simulink model "atti"  (R2022b)
settings: Solver=VariableStepAuto  StartTime=0.0  StopTime=10.0  RelTol=1e-3
values from neighbouring files (symbols this model uses):
  dt = 0.01    [attitude_main.m]
  dtheta = [x;y;z]'    [attitude_main.m]
  J = diag([0.082,0.0845,0.1377])    [attitude_main.m]
  K = lqr(sys,Q,R)    [attitude_main.m]
undefined symbols (not defined in the file or in its folder): ad, Rd, wd
libraries: shared6dof x1, aerolibutil x1
settings Model: Creator=zzy  LastModifiedBy=zzy
settings DataIOCC: ReturnWorkspaceOutputs=off

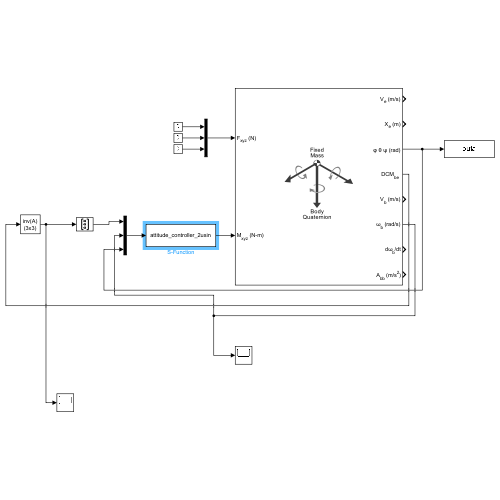
[thumbnail: Simulink's stored preview of the top-level diagram]
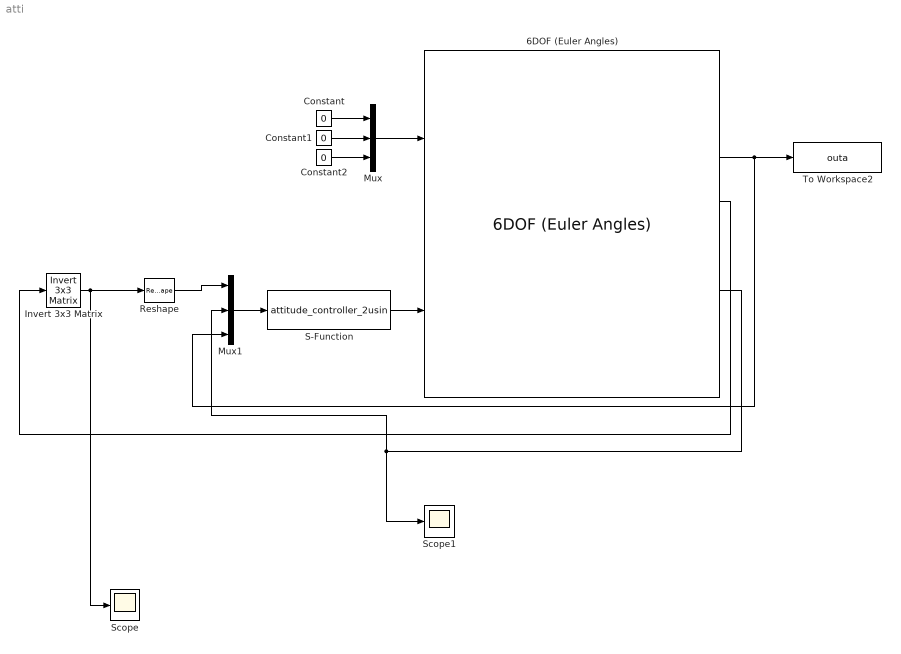
== system atti ==
  6DOF (Euler Angles) : shared6dof/6DOF (Euler Angles)  units=Metric (MKS)  mtype=Fixed  rep=Quaternion  xme_0=[0 0 0]  Vm_0=[0 0 0]  eul_0=[0 0 0]  pm_0=[0 0 0]  mass_0=1  mass_e=0.5  mass_f=2.0  inertia=J  inertia_e=eye(3)  inertia_f=2*eye(3)  k_quat=1.0  vre_flag=on  abi_flag=off  aMode=0  xme_statename=''  Vm_statename=''  eul_statename=''  quat_statename=''  pm_statename=''  mass_statename=''
  Constant : Constant  Value=0
  Constant1 : Constant  Value=0
  Constant2 : Constant  Value=0
  Invert 3x3 Matrix : aerolibutil/Invert  3x3 Matrix
  Mux : Mux  Inputs=3
  Mux1 : Mux  Inputs=3
  Reshape : Reshape  OutputDimensionality=Column vector (2-D)
  S-Function : S-Function  FunctionName=attitude_controller_2usin  Parameters=dt,Rd,wd,ad,J,K,dtheta  SFunctionDeploymentMode=off  EnableBusSupport=off
  Scope : Scope
  Scope1 : Scope
  To Workspace2 : ToWorkspace  VariableName=outa  SampleTime=-1
      settings: Save2DSignal=2-D array (concatenate along first dimension)
  wires:
  Constant1/1 -> Mux/2
  Constant/1 -> Mux/1
  Constant2/1 -> Mux/3
  Mux/1 -> 6DOF (Euler Angles)/1
  S-Function/1 -> 6DOF (Euler Angles)/2
  6DOF (Euler Angles)/6 -> Scope1/1, Mux1/2
  6DOF (Euler Angles)/4 -> Invert 3x3 Matrix/1
  Invert 3x3 Matrix/1 -> Scope/1, Reshape/1
  Mux1/1 -> S-Function/1
  Reshape/1 -> Mux1/1
  6DOF (Euler Angles)/3 -> Mux1/3, To Workspace2/1
